simulink model "polyphase_filter_demo"  (R2019b)
settings: Solver=FixedStepDiscrete  StartTime=0.0  StopTime=0.02  FixedStep=1e-6  RelTol=1e-3
libraries: dspfdesign x1, commfilt2 x1, commutil2 x1
settings Model: Creator=thomas  LastModifiedBy=thomas

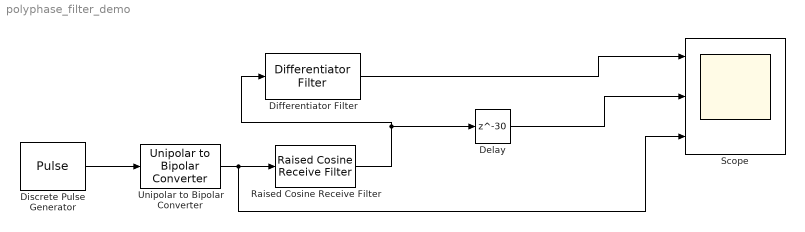
== system polyphase_filter_demo ==
  Delay : Delay  DelayLength=30  InitialCondition=0
  Differentiator Filter : dspfdesign/Differentiator Filter  DesignForMinimumOrder=on  FilterOrder=31  PassbandRipple=0.0000001  ScaleCoefficients=off  SimulateUsing=Interpreted execution  roundingMode=Floor  coeffsDataTypeStr=fixdt(1,16)
      settings: SourceProductName=DSP System Toolbox  SourceProductBaseCode=DS
  Discrete Pulse Generator : DiscretePulseGenerator  Period=4  PulseWidth=2  SampleTime=1e-6
  Raised Cosine Receive Filter : commfilt2/Raised Cosine Receive Filter  filtType=Square root  R=0.8  filtSpan=6  N=6  downFactor=1  downOffset=0  filterGain=1  InputProcessing=Columns as channels (frame based)  RateOptions=Enforce single-rate processing  framing=Mute  checkCoeff=off  variableName=rcRxFilt  currentFiltSpan=6  D=(6)/2  inputOffset=0  sampMode=Mute  saveAsFlag=0  rateMode=Downsampling  checkGain=Normalized  launchFVT=on  roundingMode=Floor  overflowMode=off  coeffDataTypeStr=Inherit: Same word length as input  coeffMin=[]  coeffMax=[]  coeffLastDataTypeStr=Inherit: Same word length as input  accumDataTypeStr=Inherit: Same as product output  accumLastDataTypeStr=Inherit: Same as product output  outputDataTypeStr=Inherit: Same as accumulator  outputMin=[]  outputMax=[]  outputLastDataTypeStr=Inherit: Same as accumulator
      settings: SourceProductName=Communications Toolbox
  Scope : Scope  NumInputPorts=3
  Unipolar to Bipolar Converter : commutil2/Unipolar to Bipolar Converter  M=2  polarity=Positive  dataType=Inherit via internal rule
      settings: SourceProductName=Communications Toolbox
  wires:
  Raised Cosine Receive Filter/1 -> Delay/1, Differentiator Filter/1
  Discrete Pulse Generator/1 -> Unipolar to Bipolar Converter/1
  Differentiator Filter/1 -> Scope/1
  Delay/1 -> Scope/2
  Unipolar to Bipolar Converter/1 -> Scope/3, Raised Cosine Receive Filter/1
